simulink model "swing_up_inv_rot_pen_sldrt_uart_com"  (R2024a)
settings: Solver=ode3  StartTime=0.0  StopTime=inf  FixedStep=Ts  RelTol=1e-3
PostLoadFcn:
  | try
  | if isempty(which('ZHAWcbfcn'));
  | callback_fid07124=fopen('ZHAWcbfcn.m','w');
  | [~]=fprintf(callback_fid07124,'%s',get_param([bdroot,'/ Setup SLDRT'],'ClipboardFcn'));
  | [~]=fclose(callback_fid07124);
  | setpref('ZHAW_SLDRT_lib','cb_fcn',which('ZHAWcbfcn'))
  | clear callback_fid07124
  | end
  | catch
  | clear callback_fid07124
  | end
  | Ts=eval(get_param([bdroot,'/ Setup SLDRT'],'Ts'));
InitFcn:
  | Ts=eval(get_param([bdroot,'/ Setup SLDRT'],'Ts'));
values from neighbouring files (symbols this model uses):
  i_max = 0.5    [inv_rot_pen_ini.m]    (also in swing_up_inv_rot_pen_ini.m)
  param = get_parameter()    [inv_rot_pen_ini.m]    (also in swing_up_inv_rot_pen_ini.m)
  Tf = 1 / (2*pi*100)    (= 0.00159154943092)    [inv_rot_pen_ini.m]    (also in swing_up_inv_rot_pen_ini.m)
  V_oben = 1 / dc_oben(1)    [swing_up_inv_rot_pen_ini.m]
  V_unten = 1 / dc_unten(1)    [swing_up_inv_rot_pen_ini.m]
undefined symbols (not defined in the file or in its folder): K_oben, K_unten, Serial_Port, Standard_Devices
libraries: sldrtlib x3, cstblocks x2
(part 2 of 2)

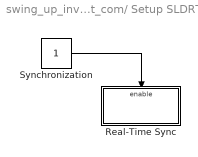
== system swing_up_inv_rot_pen_sldrt_uart_com/ Setup SLDRT ==
  Real-Time Sync : Subsystem
  Synchronization : Constant
  wires:
  Synchronization/1 -> Real-Time Sync/Enable

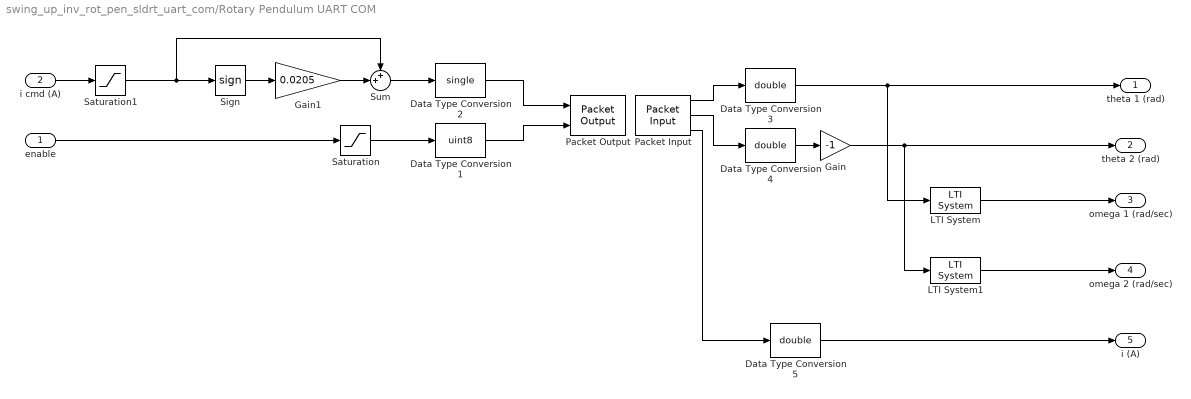
== system swing_up_inv_rot_pen_sldrt_uart_com/Rotary Pendulum UART COM ==
  enable : Inport
  i cmd (A) : Inport  Port=2
  Data Type Conversion1 : DataTypeConversion  OutDataTypeStr=uint8  SaturateOnIntegerOverflow=off  RndMeth=Floor
  Data Type Conversion2 : DataTypeConversion  OutDataTypeStr=single  SaturateOnIntegerOverflow=off  RndMeth=Floor
  Data Type Conversion3 : DataTypeConversion  OutDataTypeStr=double  SaturateOnIntegerOverflow=off  RndMeth=Floor
  Data Type Conversion4 : DataTypeConversion  OutDataTypeStr=double  SaturateOnIntegerOverflow=off  RndMeth=Floor
  Data Type Conversion5 : DataTypeConversion  OutDataTypeStr=double  SaturateOnIntegerOverflow=off  RndMeth=Floor
  Gain : Gain  Gain=-1
  Gain1 : Gain  Gain=0.0205
  LTI System : cstblocks/LTI System  sys=G_diff  IC=[]  PadeOrder=0
  LTI System1 : cstblocks/LTI System  sys=G_diff  IC=[]  PadeOrder=0
  Packet Input : sldrtlib/Packet Input  SampleTime=Ts  MaxMissedTicks=10  ShowMissedTicks=off  YieldWhenWaiting=off  DrvName=Standard_Devices/Serial_Port  DrvAddress=8  DrvOptions=[115200 8 0 0 0 0 0 0]  PacketSize=4 + 4 + 4  DataTypes={'single', 'single', 'single'}  ShowReady=off  ShowError=off  PacketID=1  ByteOrder=1  ShowTimestamp=off
      settings: AttributesFormatString=Serial Port [8]
  Packet Output : sldrtlib/Packet Output  SampleTime=Ts  MaxMissedTicks=10  ShowMissedTicks=off  YieldWhenWaiting=off  DrvName=Standard_Devices/Serial_Port  DrvAddress=8  DrvOptions=[115200 8 0 0 0 0 0 0]  PacketSize=4 + 1  DataTypes={'single', 'uint8'}  ShowReady=off  ShowError=off  PacketID=1  ByteOrder=1  InitialValue=[]  FinalValue=[]
      settings: AttributesFormatString=Serial Port [8]
  Saturation : Saturate  UpperLimit=1.0  LowerLimit=0.0
  Saturation1 : Saturate  UpperLimit=i_max  LowerLimit=-i_max
  Sign : Signum
  Sum : Sum  Inputs=++|
  theta 1 (rad) : Outport
  theta 2 (rad) : Outport  Port=2
  omega 1 (rad/sec) : Outport  Port=3
  omega 2 (rad/sec) : Outport  Port=4
  i (A) : Outport  Port=5
  wires:
  Data Type Conversion2/1 -> Packet Output/1
  Packet Input/2 -> Data Type Conversion4/1
  Saturation/1 -> Data Type Conversion1/1
  Packet Input/1 -> Data Type Conversion3/1
  Data Type Conversion1/1 -> Packet Output/2
  enable/1 -> Saturation/1
  Data Type Conversion3/1 -> LTI System/1, theta 1 (rad)/1
  Data Type Conversion4/1 -> Gain/1
  LTI System/1 -> omega 1 (rad/sec)/1
  LTI System1/1 -> omega 2 (rad/sec)/1
  Gain/1 -> LTI System1/1, theta 2 (rad)/1
  Packet Input/3 -> Data Type Conversion5/1
  Data Type Conversion5/1 -> i (A)/1
  Sign/1 -> Gain1/1
  Gain1/1 -> Sum/2
  i cmd (A)/1 -> Saturation1/1
  Sum/1 -> Data Type Conversion2/1
  Saturation1/1 -> Sum/1, Sign/1

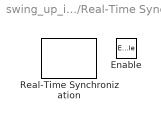
== system swing_up_inv_rot_pen_sldrt_uart_com/ Setup SLDRT/Real-Time Sync ==
  Enable : EnablePort
  Real-Time Synchronization : sldrtlib/Real-Time Synchronization  SampleTime=Ts  MaxMissedTicks=inf  ShowMissedTicks=off  YieldWhenWaiting=off

== matlab function swing_up_inv_rot_pen_sldrt_uart_com/Controller ==
  settings: updateMethod=DISCRETE  sampleTime=Ts
  data theta_2 settings: description=(rad)
  data: theta_1 input; theta_2 input; i output size=1; param parameter; k input; switch_angle input; switch_position input; K_oben parameter; K_unten parameter; Ts parameter; Tf parameter; states output; E output; u_acc output; omega1_soll input; V_unten parameter; V_oben parameter
function [i, states, E, u_acc] = fcn(theta_1, theta_2, param, k, switch_angle, switch_position, K_oben, K_unten, Ts, Tf, omega1_soll, V_unten, V_oben)

    % Persistente Variablen für Zustände und Filter
    persistent mode theta_1_offset r_soll
    if isempty(mode)
        mode = 0;  % Start im Modus 0: unten regeln
        theta_1_offset = 0;
        r_soll = 0;
    end

    % Initialisierung für Coder
    i = 0;
    states = zeros(4,1); 
    E = 0;
    u_acc = 0;
    

    % Filterung der Winkelgeschwindigkeit
    [omega_1f, omega_2f] = filter_velocity(theta_1, theta_2, Ts, Tf);

    % Normierter Winkel für obenregelung (theta_2_up = 0 wenn oben)
    theta_2_up = abs(mod(theta_2, 2*pi) - pi);

    % Geschwindigkeitsvorgabe Motor
    r_soll = velocity_control_motor(r_soll, omega1_soll, Ts);

   switch mode
    case 0  % Unten regeln
        theta_2_short = atan2(sin(theta_2), cos(theta_2));
        states = [theta_1-theta_1_offset; theta_2_short; omega_1f; omega_2f];

        if switch_position == 1
            mode = 1;  % Wechsel zu Aufschwingen
        elseif theta_2_up >= 90 * pi / 180
            i = (r_soll*V_unten) - K_unten * states;
            % disp('Regeln unten');
        else
            i = 0;
            theta_1_offset = theta_1;
            r_soll = 0;
            % disp('Abschwingen');
        end

    case 1  % Aufschwingen
        % Energie Berechnung für Aufschwingen
        [i, E, u_acc] = calc_upswing(theta_2, omega_2f, omega_1f, param, k);
        theta_2_short = atan2(sin(theta_2 + pi), cos(theta_2 + pi));
        states = [theta_1; theta_2_short; omega_1f; omega_2f];
        % disp('Aufschwingen');
        if switch_position > 0 && theta_2_up <= switch_angle * pi / 180
            mode = 2;  % Umschalten auf oben regeln
            theta_1_offset = theta_1;
            r_soll = 0;
        end
        if switch_position == 0
            mode = 0;  % Umschalten auf abschwingen / unten regelen
        end

    case 2  % Oben regeln   
        theta_2_short = atan2(sin(theta_2 + pi), cos(theta_2+ pi));
        states = [theta_1-theta_1_offset; theta_2_short; omega_1f; omega_2f];
        i = r_soll * V_oben - K_oben * states;
        % disp('Regeln oben');

        if theta_2_up > switch_angle * pi / 180
            mode = 1; % Umschalten auf Aufschwingen
        end

        if switch_position == 0 
            mode = 0;  % Umschalten auf abschwingen / unten regeln
        end

    case 3 % Geschwindigkeits Überschreitung
           theta_2_short = atan2(sin(theta_2), cos(theta_2));
           states = [theta_1-theta_1_offset; theta_2_short; omega_1f; omega_2f];
           i = 0;

   end

    % Kompensation der Haftreibung
    i = sign(i)*0.0205+i;

    % Begrenzung Motor
    [mode, i] = motor_limit(param, omega_1f, i, mode);
    
end

function [omega_1f, omega_2f] = filter_velocity(theta_1, theta_2, Ts, Tf_sim)
    persistent theta_1_past theta_2_past omega_1f_past omega_2f_past a b
    if isempty(theta_1_past)
        theta_1_past = theta_1;
        theta_2_past = theta_2;
        omega_1f_past = 0;
        omega_2f_past = 0;
        b = 2.0 / (2*Tf_sim + Ts);
        a = (Ts - 2*Tf_sim) / (2*Tf_sim + Ts);
    end

    omega_1f = b * (theta_1 - theta_1_past) - a * omega_1f_past;
    omega_2f = b * (theta_2 - theta_2_past) - a * omega_2f_past;

    theta_1_past = theta_1;
    theta_2_past = theta_2;
    omega_1f_past = omega_1f;
    omega_2f_past = omega_2f;
end

function [i, E, u_acc] = calc_upswing(theta_2, omega_2f, omega_1f, param, k)
    persistent J J_arm Er
    if isempty(J)
        J = param.m2 * param.L2^2 / 12; % Trägheitmoment des Pendels
        J_arm = param.J1zz;
        Er = 2 * param.m2 * param.g * param.l2;
    end

    E = 0.5 * J * omega_2f^2 + param.m2 * -param.g * param.l2 * (cos(theta_2)-1);
    u_acc = k * (E - Er) * sign(omega_2f * cos(theta_2));  % Energie-Regelung
    % u = u_acc * param.m1 * param.L1 * param.Rm / param.kt; % Spannungsberechnung wie bei Quanser
    i = (u_acc / param.L1) * J_arm / param.km - 0.005*omega_1f;
end

function [mode, i] = motor_limit(param, omega_1f, i, mode)
    %Geschwindigkeitsbegrenzung Motor
    if abs(omega_1f) > 35
        mode = 3;
    end
    % Begrenzung auf ±1A
    i = min(max(i, -param.i_max_setpoint), param.i_max_setpoint);
end

function r_soll = velocity_control_motor(r_soll, omega1_soll, Ts)
    % Mindesgestgeschwindigkeit Slider Motor
    if abs(omega1_soll) < 0.15
        omega1_soll = 0;
    end
    % Saturation auf max 1 U/s
    omega1_sat = min(max(omega1_soll, -2*pi), 2*pi);
    r_soll = Ts*(omega1_sat) + r_soll;
end
